simulink model "vpToVsOpen"  (R2024b)
settings: Solver=ode15s  StartTime=0.0  StopTime=10.0  MaxStep=0.2  RelTol=1e-3
values from neighbouring files (symbols this model uses):
  den = [coeff3, coeff2, coeff1, 0]    [initParams.m]
  num = [-1]    [initParams.m]
settings Model: Creator=steve0gillet  LastModifiedBy=steve0gillet
settings DebuggingCC: ReadBeforeWriteMsg=DisableAll  WriteAfterWriteMsg=DisableAll  WriteAfterReadMsg=DisableAll  MultiTaskDSMMsg=none
settings ModelReferenceCC: UpdateModelReferenceTargets=IfOutOfDate
settings SFSimCC: SFSimEcho=off

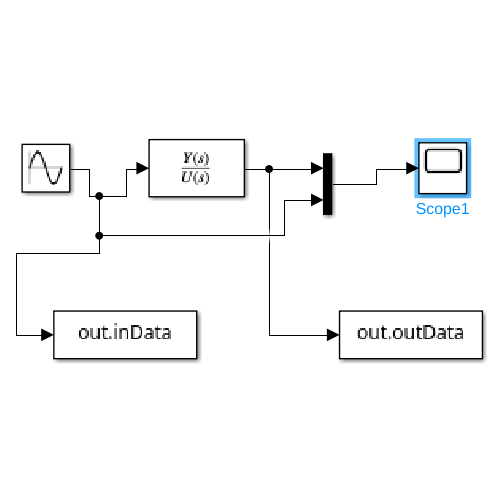
[thumbnail: Simulink's stored preview of the top-level diagram]
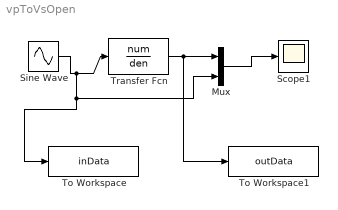
== system vpToVsOpen ==
  Mux : Mux  Inputs=2
  Scope1 : Scope
  Sine Wave : Sin  Frequency=pi*2  SampleTime=0
  To Workspace : ToWorkspace  VariableName=inData  SaveFormat=Timeseries  SampleTime=-1
  To Workspace1 : ToWorkspace  VariableName=outData  SaveFormat=Timeseries  SampleTime=-1
  Transfer Fcn : TransferFcn  Numerator=num  Denominator=den
  wires:
  Sine Wave/1 -> To Workspace/1, Mux/2, Transfer Fcn/1
  Transfer Fcn/1 -> To Workspace1/1, Mux/1
  Mux/1 -> Scope1/1
